simulink model "PID"  (R2020a)
settings: Solver=ode14x  StartTime=0.0  StopTime=15  FixedStep=1e-3  RelTol=1e-3
values from neighbouring files (symbols this model uses):
  new_kd = gains(1)    [script.m]    (also in script_pid.m)
  new_ki = gains(3)    [script.m]    (also in script_pid.m)
  new_kp = gains(2)    [script.m]    (also in script_pid.m)
settings Model: Creator=Admin  LastModifiedBy=Admin
settings DataIOCC: ReturnWorkspaceOutputsName=out_ffw

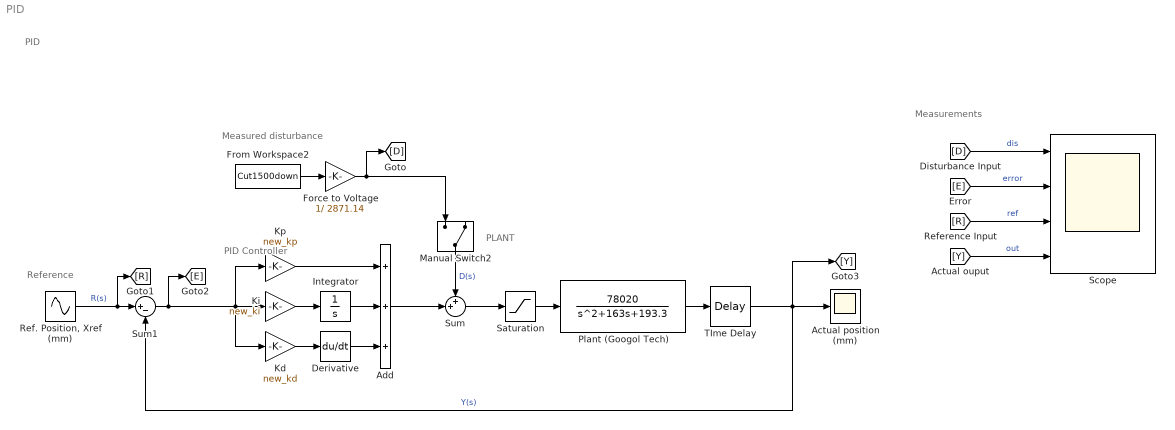
== system PID ==
  note: PID
  note: Measured disturbance
  note: PID Controller
  note: PLANT
  note: Measurements
  note: Reference
  Actual position (mm) : Scope
  Add : Sum  Inputs=+++
  Derivative : Derivative
  Force to Voltage : Gain  Gain=1/ 2871.14
  From Workspace2 : FromWorkspace  VariableName=Cut1500down  OutDataTypeStr=double  OutputAfterFinalValue=Setting to zero
  Integrator : Integrator
  Kd : Gain  Gain=new_kd
  Ki : Gain  Gain=new_ki
  Kp : Gain  Gain=new_kp
  Manual Switch2 : ManualSwitch  CurrentSetting=0
  Plant (Googol Tech) : TransferFcn  Numerator=[78020]  Denominator=[1 163 193.3]
  "Ref. Position, Xref (mm)" : Sin  Amplitude=5  Frequency=0.5*(2*pi)  SampleTime=0  Offset=1/2000
  Saturation : Saturate  UpperLimit=92  LowerLimit=-92
  Scope : Scope  NumInputPorts=4
  Sum : Sum  Inputs=++|
  Sum1 : Sum  Inputs=|+-
  TIme Delay : TransportDelay  DelayTime=0.0012
  wires:
  Sum/1 -> Saturation/1
  Saturation/1 -> Plant (Googol Tech)/1
  Kd/1 -> Derivative/1
  Manual Switch2/1 -> Sum/1  "D(s)"
  [D] -> Scope/1  "dis"
  [Y] -> Scope/4  "out"
  Plant (Googol Tech)/1 -> TIme Delay/1
  Derivative/1 -> Add/3
  [R] -> Scope/3  "ref"
  Sum1/1 -> Kd/1, Ki/1, Kp/1, [E]
  Add/1 -> Sum/2
  [E] -> Scope/2  "error"
  Integrator/1 -> Add/2
  "Ref. Position, Xref (mm)"/1 -> [R], Sum1/1  "R(s)"
  TIme Delay/1 -> Actual position (mm)/1, [Y], Sum1/2  "Y(s)"
  Force to Voltage/1 -> Manual Switch2/1, [D]
  Ki/1 -> Integrator/1
  Kp/1 -> Add/1
  From Workspace2/1 -> Force to Voltage/1
